simulink model "sistema_finale_ciclo_chiuso"  (R2023b)
settings: Solver=VariableStepAuto  StartTime=0.0  StopTime=10.0  RelTol=1e-3
undefined symbols (not defined in the file): Tc
libraries: cstblocks x2
settings Model: Creator=USER  LastModifiedBy=Pasquale
settings SolverCC: AlgebraicLoopSolver=TrustRegion
settings OptimizationCC: ReuseModelBlockBuffer=off
settings DebuggingCC: UnconnectedInputMsg=warning  UnconnectedOutputMsg=warning  UnconnectedLineMsg=warning
settings ModelReferenceCC: EnableRefExpFcnMdlSchedulingChecks=on
settings RTWCC: DLArmComputeVersion=19.05

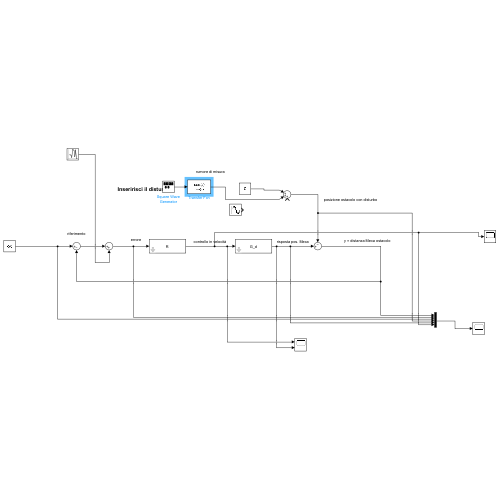
[thumbnail: Simulink's stored preview of the top-level diagram]
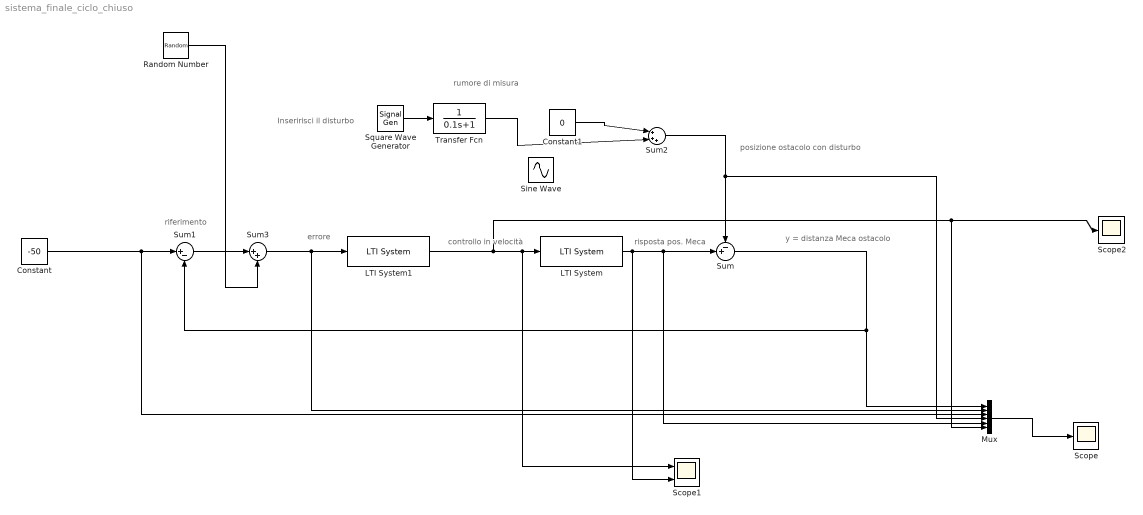
== system sistema_finale_ciclo_chiuso ==
  note: rumore di misura
  note: Inseririsci il disturbo
  note: y = distanza Meca ostacolo
  note: posizione ostacolo con disturbo
  note: risposta pos. Meca
  note: controllo in velocità
  note: errore
  note: riferimento
  Constant : Constant  Value=-50
  Constant1 : Constant  Value=0
  LTI System : cstblocks/LTI System  sys=G_d  IC=[]  PadeOrder=0
  LTI System1 : cstblocks/LTI System  sys=R  IC=[]  PadeOrder=0
  Mux : Mux  Inputs=6
  Random Number : RandomNumber  Variance=1.5  SampleTime=Tc
  Scope : Scope
  Scope1 : Scope  NumInputPorts=2
  Scope2 : Scope
  Sine Wave : Sin  Amplitude=10  Frequency=5  SampleTime=Tc
  Square Wave Generator : SignalGenerator  WaveForm=square  Amplitude=50  Frequency=0.25
  Sum : Sum  Inputs=-+|
  Sum1 : Sum  Inputs=|+-
  Sum2 : Sum  Inputs=|+++
  Sum3 : Sum  Inputs=|++
  Transfer Fcn : TransferFcn  Denominator=[0.1 1]
  wires:
  LTI System1/1 -> Mux/6, Scope2/1, Scope1/1, LTI System/1
  LTI System/1 -> Scope1/2, Mux/5, Sum/2
  Sum/1 -> Sum1/2, Mux/1
  Constant/1 -> Sum1/1, Mux/3
  Mux/1 -> Scope/1
  Constant1/1 -> Sum2/1
  Sum2/1 -> Sum/1, Mux/4
  Sum1/1 -> Sum3/1
  Sum3/1 -> Mux/2, LTI System1/1
  Random Number/1 -> Sum3/2
  Square Wave Generator/1 -> Transfer Fcn/1
  Transfer Fcn/1 -> Sum2/2
